simulink model "SIMU_TANKS"  (R2017b)
settings: Solver=VariableStepAuto  StartTime=0.0  StopTime=40  RelTol=1e-3
settings Model: Creator=Jahaira  LastModifiedBy=Jahaira

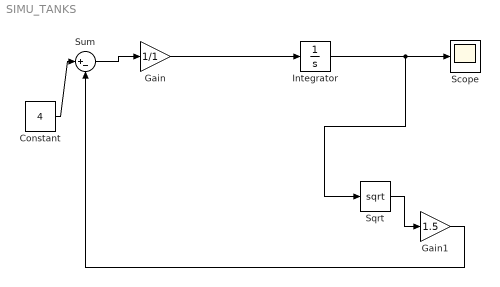
== system SIMU_TANKS ==
  Constant : Constant  Value=4
  Gain : Gain  Gain=1/1
  Gain1 : Gain  Gain=1.5
  Integrator : Integrator
  Scope : Scope
  Sqrt : Sqrt  SaturateOnIntegerOverflow=on
  Sum : Sum  Inputs=|+-
  wires:
  Constant/1 -> Sum/1
  Sum/1 -> Gain/1
  Gain/1 -> Integrator/1
  Integrator/1 -> Sqrt/1, Scope/1
  Sqrt/1 -> Gain1/1
  Gain1/1 -> Sum/2
